simulink model "K2_change_control_signal"  (R2021a)
settings: Solver=FixedStepAuto  StartTime=0.0  StopTime=15  FixedStep=0.01  RelTol=1e-3
libraries: fuzblock x4
settings Model: Creator=Admin  LastModifiedBy=Admin

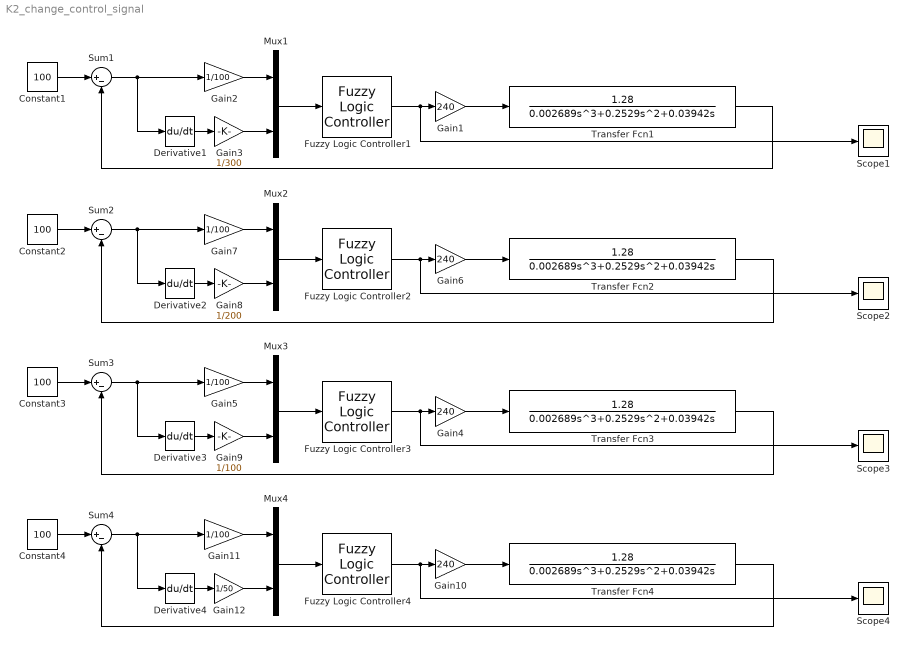
== system K2_change_control_signal ==
  Constant{1..4} (4 alike) : Constant  Value=100
  Derivative{1..4} (4 alike) : Derivative
  Fuzzy Logic Controller{1..4} (4 alike) : fuzblock/Fuzzy Logic  Controller  FIS='Rules_fuzzy_week6.fis'  OutputSampleNumber=101  DataType=double  FuzzifiedInputs=off  RuleFiringStrengths=off  RuleOutputs=off  AggregatedOutputs=off  SimulateUsing=Interpreted execution  OutOfRangeInputValueMessage=warning  NoRuleFiredMessage=warning  EmptyOutputFuzzySetMessage=warning
  Gain{1,4,6,10} (4 alike) : Gain  Gain=240
  Gain{2,5,7,9,11} (5 alike) : Gain  Gain=1/100
  Gain12 : Gain  Gain=1/50
  Gain3 : Gain  Gain=1/300
  Gain8 : Gain  Gain=1/200
  Mux{1..4} (4 alike) : Mux  Inputs=2
  Scope{1..4} (4 alike) : Scope
  Sum{1..4} (4 alike) : Sum  Inputs=|+-
  Transfer Fcn{1..4} (4 alike) : TransferFcn  Numerator=[1.28]  Denominator=[0.002689 0.2529 0.03942 0]
  wires:
  Transfer Fcn3/1 -> Sum3/2
  Fuzzy Logic Controller4/1 -> Scope4/1, Gain10/1
  Constant4/1 -> Sum4/1
  Constant3/1 -> Sum3/1
  Gain11/1 -> Mux4/1
  Mux4/1 -> Fuzzy Logic Controller4/1
  Sum4/1 -> Derivative4/1, Gain11/1
  Gain9/1 -> Mux3/2
  Gain5/1 -> Mux3/1
  Fuzzy Logic Controller3/1 -> Scope3/1, Gain4/1
  Transfer Fcn4/1 -> Sum4/2
  Derivative4/1 -> Gain12/1
  Gain12/1 -> Mux4/2
  Mux1/1 -> Fuzzy Logic Controller1/1
  Gain4/1 -> Transfer Fcn3/1
  Sum1/1 -> Derivative1/1, Gain2/1
  Transfer Fcn1/1 -> Sum1/2
  Derivative1/1 -> Gain3/1
  Mux3/1 -> Fuzzy Logic Controller3/1
  Gain3/1 -> Mux1/2
  Gain2/1 -> Mux1/1
  Derivative3/1 -> Gain9/1
  Mux2/1 -> Fuzzy Logic Controller2/1
  Transfer Fcn2/1 -> Sum2/2
  Gain8/1 -> Mux2/2
  Gain7/1 -> Mux2/1
  Sum2/1 -> Derivative2/1, Gain7/1
  Fuzzy Logic Controller1/1 -> Scope1/1, Gain1/1
  Sum3/1 -> Derivative3/1, Gain5/1
  Fuzzy Logic Controller2/1 -> Scope2/1, Gain6/1
  Derivative2/1 -> Gain8/1
  Gain10/1 -> Transfer Fcn4/1
  Constant1/1 -> Sum1/1
  Constant2/1 -> Sum2/1
  Gain6/1 -> Transfer Fcn2/1
  Gain1/1 -> Transfer Fcn1/1
